simulink model "sensor_fusion"  (R2026a)
settings: Solver=ode1  StopTime=inf  FixedStep=1/60  EnableMultiTasking=on
model workspace (MAT data in the model file):
  downCamStepSize = Simulink.Parameter
  downCamStepSize.Value = Simulink.data.Expression
  downCamStepSize.Value.ExpressionString = "qc_get_step_size*ceil(1/60/qc_get_step_size)"
  downCamStepSize.Complexity = 'real'
  downCamStepSize.Dimensions = -1
  downCamStepSize.DataType = 'auto'
  lidarStepSize = Simulink.Parameter
  lidarStepSize.Value = Simulink.data.Expression
  lidarStepSize.Value.ExpressionString = "qc_get_step_size*ceil(1/5/qc_get_step_size)"
  lidarStepSize.Complexity = 'real'
  lidarStepSize.Dimensions = -1
  lidarStepSize.DataType = 'auto'
  mainStepSize = Simulink.Parameter
  mainStepSize.Value = Simulink.data.Expression
  mainStepSize.Value.ExpressionString = "qc_get_step_size"
  mainStepSize.Complexity = 'real'
  mainStepSize.Dimensions = -1
  mainStepSize.DataType = 'auto'
  mode = Simulink.Parameter
  mode.Value = 1
  mode.Complexity = 'real'
  mode.Dimensions = [1 1]
  mode.Description = '0 - education speeds via wheel speed commands
    | 1 - education speeds via body speed commands
    | 2 - research speeds via wheel speed commands
    | 3 - research speeds via body speed commands'
  mode.DataType = 'auto'
  realSenseStepSize = Simulink.Parameter
  realSenseStepSize.Value = Simulink.data.Expression
  realSenseStepSize.Value.ExpressionString = "qc_get_step_size*ceil(1/30/qc_get_step_size)"
  realSenseStepSize.Complexity = 'real'
  realSenseStepSize.Dimensions = -1
  realSenseStepSize.DataType = 'auto'
undefined symbols (not defined in the file): Point
libraries: quarc_library x21, simulink x2
settings Model: SimulationMode=external  ExtModeTrigDuration=10000  Creator=mbohra  LastModifiedBy=rdu
settings SolverCC: PositivePriorityOrder=on
settings DebuggingCC: ParameterPrecisionLossMsg=none
settings HardwareCC: ProdBitPerLong=64.0  ProdLargestAtomicInteger=LongLong  ProdLargestAtomicFloat=Double  ProdHWDeviceType=ARM Compatible->ARM 64-bit (LP64)
settings RTWCC: SystemTargetFile=quarc_linux_qbot_platform.tlc  TemplateMakefile=quarc_default_tmf  Toolchain=QUARC linux_qbot_platform | gmake (64-bit Windows)  BuildConfiguration=Faster Runs  Description=QUARC Linux QBot Platform Target Using Toolchain
settings STFCustomTargetCC: SystemTargetFile=quarc_linux_qbot_platform.tlc  MultiwordLength=2048.0  ConcurrentExecutionCompliant=on  UseToolchainInfoCompliant=on  StripSymbols=off  MinimumThreadPriority=20.0
settings GRTTargetCC: ExtMode=on  ExtModeMexFile=quarc_comm  ExtModeMexArgs='-w -d /tmp -uri %u','tcpip://192.168.5.3:17001'  ParMdlRefBuildCompliant=off  CompOptLevelCompliant=off  CombineOutputUpdateFcns=off  MatFileLogging=off  CPPClassGenCompliant=off  GRTInterface=on
settings ConfigComp: CovMetricSettings=dswe

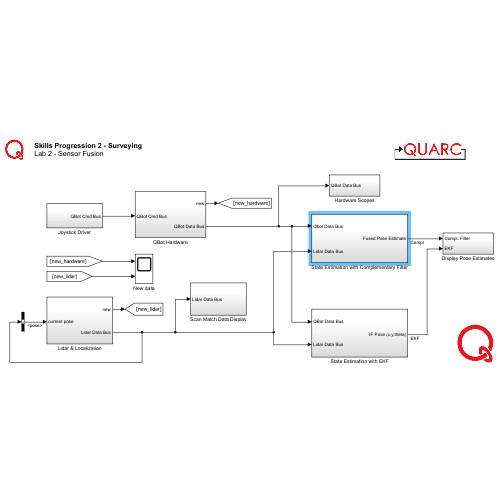
[thumbnail: Simulink's stored preview of the top-level diagram]
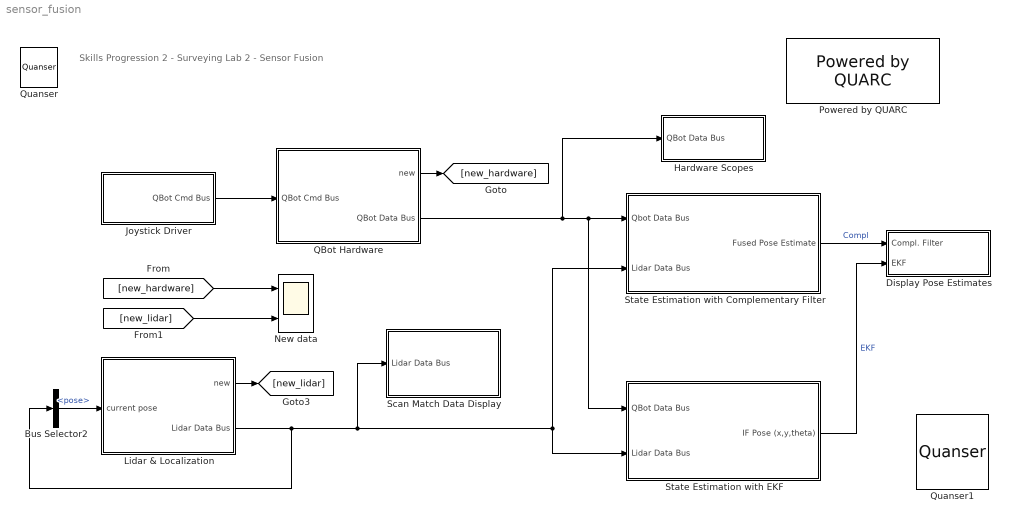
== system sensor_fusion ==
  note: Skills Progression 2 - Surveying
      | Lab 2 - Sensor Fusion
  Bus Selector2 : BusSelector  OutputSignals=pose
  Display Pose Estimates : Subsystem
  Hardware Scopes : Subsystem
  Joystick Driver : Subsystem
  Lidar & Localization : Subsystem
  New data : Scope  NumInputPorts=2
      settings: Title=Hardware Data New?  ActiveDisplayYMinimum=0.9  ActiveDisplayYMaximum=1.1  DataLoggingDecimation=10  DataLoggingVariableName=ScopeData2
  Powered by QUARC : quarc_library/Logos/Powered by QUARC
  QBot Hardware : Subsystem
  Quanser : quarc_library/Logos/Quanser
  Quanser1 : quarc_library/Logos/Quanser
  Scan Match Data Display : Subsystem
  State Estimation with Complementary Filter : Subsystem
  State Estimation with EKF : Subsystem
  wires:
  QBot Hardware/1(new) -> [new_hardware]
  Lidar & Localization/1(new) -> [new_lidar]
  [new_lidar] -> New data/2
  [new_hardware] -> New data/1
  Bus Selector2/1 -> Lidar & Localization/1(current pose)  "<pose>"
  Lidar & Localization/2(Lidar Data Bus) -> State Estimation with EKF/2(Lidar Data Bus), State Estimation with Complementary Filter/2(Lidar Data Bus), Scan Match Data Display/1(Lidar Data Bus), Bus Selector2/1
  Joystick Driver/1(QBot Cmd Bus) -> QBot Hardware/1(QBot Cmd Bus)
  QBot Hardware/2(QBot Data Bus) -> State Estimation with Complementary Filter/1(Qbot Data Bus), State Estimation with EKF/1(QBot Data Bus), Hardware Scopes/1(QBot Data Bus)
  State Estimation with Complementary Filter/1(Fused Pose Estimate) -> Display Pose Estimates/1(Compl. Filter)  "Compl"
  State Estimation with EKF/1(IF Pose (x,y,theta)) -> Display Pose Estimates/2(EKF)  "EKF"

== system sensor_fusion/Display Pose Estimates ==
  Compl. Filter : Inport
  EKF : Inport  Port=2
  Mux : Mux  Inputs=2
  Mux1 : Mux  Inputs=2
  Mux2 : Mux  Inputs=2
  "Pose Estimates " : Scope  NumInputPorts=3
      settings: ActiveDisplayString=3  Title=Theta (rad)  ActiveDisplayYMinimum=-3.7845885644041823  ActiveDisplayYMaximum=8.5346333601811839  DataLoggingVariableName=ScopeData4
  Selector : Selector  InputPortWidth=3  IndexOptions=Index vector (dialog)  Indices=[1]  OutputSizes=1
  Selector1 : Selector  InputPortWidth=3  IndexOptions=Index vector (dialog)  Indices=[1]  OutputSizes=1
  Selector2 : Selector  InputPortWidth=3  IndexOptions=Index vector (dialog)  Indices=[2]  OutputSizes=1
  Selector3 : Selector  InputPortWidth=3  IndexOptions=Index vector (dialog)  Indices=[2]  OutputSizes=1
  Selector4 : Selector  InputPortWidth=3  IndexOptions=Index vector (dialog)  Indices=[3]  OutputSizes=1
  Selector5 : Selector  InputPortWidth=3  IndexOptions=Index vector (dialog)  Indices=[3]  OutputSizes=1
  wires:
  Compl. Filter/1 -> Selector4/1, Selector2/1, Selector/1
  Mux/1 -> "Pose Estimates "/1
  Selector/1 -> Mux/1  "Compl"
  EKF/1 -> Selector5/1, Selector3/1, Selector1/1
  Selector1/1 -> Mux/2  "EKF"
  Selector2/1 -> Mux1/1  "Compl"
  Selector3/1 -> Mux1/2  "EKF"
  Selector5/1 -> Mux2/2  "EKF"
  Selector4/1 -> Mux2/1  "Compl"
  Mux1/1 -> "Pose Estimates "/2
  Mux2/1 -> "Pose Estimates "/3

== system sensor_fusion/Hardware Scopes ==
  QBot Data Bus : Inport
  Accelerometer : Scope  Commented=on
      settings: ActiveDisplayYMinimum=-1.32758  ActiveDisplayYMaximum=11.23  DataLoggingVariableName=ScopeData9
  Battery Sense : Scope  Commented=on
      settings: ActiveDisplayYMinimum=12.81161  ActiveDisplayYMaximum=12.96349  DataLoggingVariableName=ScopeData10
  Bus Selector : BusSelector  OutputSignals=Wheel position (rad) [2],Wheel Speeds (rad/s) [2],Motor Cmd (Volts) [2],Acceleration (m/s/s) [3],Gyroscope (rad/s) [3],Current (Amps) [2],Battery (Volts)
  Cmd Voltage : Scope  Commented=on
      settings: ActiveDisplayYMinimum=-1  ActiveDisplayYMaximum=1  DataLoggingVariableName=ScopeData11
  Current Sense : Scope  Commented=on
      settings: ActiveDisplayYMinimum=-0.05029  ActiveDisplayYMaximum=0.45265  DataLoggingVariableName=ScopeData12
  Encoder : Scope  Commented=on
      settings: ActiveDisplayYMinimum=-23.46955  ActiveDisplayYMaximum=23.65434  DataLoggingVariableName=ScopeData13
  Gyroscope : Scope  Commented=on
      settings: ActiveDisplayYMinimum=-0.40322  ActiveDisplayYMaximum=1.99912  DataLoggingVariableName=ScopeData14
  Tachometer : Scope  Commented=on
      settings: ActiveDisplayYMinimum=-11.69986  ActiveDisplayYMaximum=11.67552  DataLoggingVariableName=ScopeData15
  wires:
  Bus Selector/6 -> Current Sense/1  "<Current (Amps) [2]>"
  QBot Data Bus/1 -> Bus Selector/1
  Bus Selector/3 -> Cmd Voltage/1  "<Motor Cmd (Volts) [2]>"
  Bus Selector/7 -> Battery Sense/1  "<Battery (Volts)>"
  Bus Selector/4 -> Accelerometer/1  "<Acceleration (m/s/s) [3]>"
  Bus Selector/1 -> Encoder/1  "<Wheel position (rad) [2]>"
  Bus Selector/2 -> Tachometer/1  "<Wheel Speeds (rad/s) [2]>"
  Bus Selector/5 -> Gyroscope/1  "<Gyroscope (rad/s) [3]>"

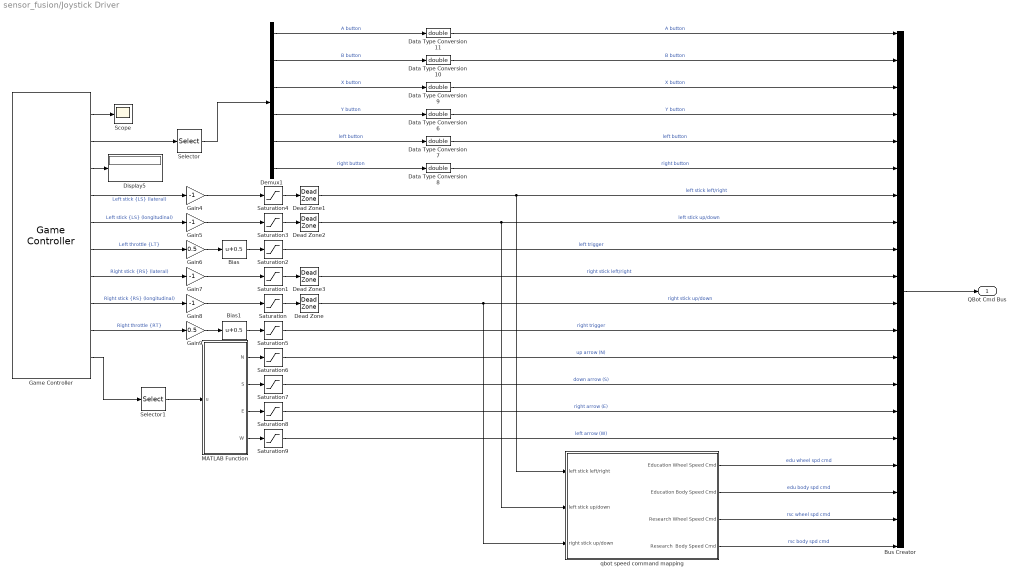
== system sensor_fusion/Joystick Driver ==
  Bias : Bias  Bias=0.5  SaturateOnIntegerOverflow=off
  Bias1 : Bias  Bias=0.5  SaturateOnIntegerOverflow=off
  Bus Creator : BusCreator  Inputs=20
  Data Type Conversion{6..11} (6 alike) : DataTypeConversion  OutDataTypeStr=double  SaturateOnIntegerOverflow=off  RndMeth=Floor
  Dead Zone{,1..3} (4 alike) : DeadZone  LowerValue=-0.05  UpperValue=0.05
  Demux1 : Demux  Outputs=6
  Display5 : Display
  Gain{4..5,7..8} (4 alike) : Gain  Gain=-1
  Gain6 : Gain  Gain=0.5
  Gain9 : Gain  Gain=0.5
  Game Controller : quarc_library/Devices/Peripherals/Target/Game Controller  controller=1  buffer_size=12  deadzone=[]  saturation=[]  sample_time=qc_get_step_size  auto_center=off  enabled=on
      settings: SourceProductName=QUARC Targets
  MATLAB Function : MATLAB Function  TreatAsAtomicUnit=on
  Saturation{,1,3..4} (4 alike) : Saturate  UpperLimit=1  LowerLimit=-1
  Saturation{2,5..9} (6 alike) : Saturate  UpperLimit=1  LowerLimit=0
  Scope : Scope
      settings: ActiveDisplayYMinimum=-1  ActiveDisplayYMaximum=1
  Selector : Selector  InputPortWidth=32  IndexOptions=Index vector (dialog)  Indices=[1:6]  OutputSizes=1
  Selector1 : Selector  InputPortWidth=4  IndexOptions=Index vector (dialog)  Indices=1  OutputSizes=1
  qbot speed command mapping : Subsystem
  QBot Cmd Bus : Outport
  wires:
  Game Controller/1 -> Scope/1
  Game Controller/2 -> Selector/1
  Game Controller/3 -> Display5/1
  Game Controller/4 -> Gain4/1  "Left stick {LS} (lateral)"
  Game Controller/5 -> Gain5/1  "Left stick {LS} (longitudinal)"
  Game Controller/6 -> Gain6/1  "Left throttle {LT}"
  Game Controller/7 -> Gain7/1  "Right stick {RS} (lateral)"
  Game Controller/8 -> Gain8/1  "Right stick {RS} (longitudinal)"
  Game Controller/9 -> Gain9/1  "Right throttle {RT}"
  Game Controller/10 -> Selector1/1
  Selector/1 -> Demux1/1
  Selector1/1 -> MATLAB Function/1(u)
  Gain6/1 -> Bias/1
  Gain9/1 -> Bias1/1
  Gain8/1 -> Saturation/1
  Gain7/1 -> Saturation1/1
  Gain5/1 -> Saturation3/1
  Gain4/1 -> Saturation4/1
  Bias/1 -> Saturation2/1
  Bias1/1 -> Saturation5/1
  Saturation4/1 -> Dead Zone1/1
  Saturation3/1 -> Dead Zone2/1
  Saturation1/1 -> Dead Zone3/1
  Saturation/1 -> Dead Zone/1
  MATLAB Function/1(N) -> Saturation6/1
  MATLAB Function/2(S) -> Saturation7/1
  MATLAB Function/3(E) -> Saturation8/1
  MATLAB Function/4(W) -> Saturation9/1
  Demux1/5 -> Data Type Conversion7/1  "left button"
  Demux1/6 -> Data Type Conversion8/1  "right button"
  Dead Zone/1 -> qbot speed command mapping/3(right stick up/down), Bus Creator/11  "right stick up/down"
  Dead Zone1/1 -> qbot speed command mapping/1(left stick left/right), Bus Creator/7  "left stick left/right"
  Demux1/4 -> Data Type Conversion6/1  "Y button"
  Demux1/3 -> Data Type Conversion9/1  "X button"
  Demux1/2 -> Data Type Conversion10/1  "B button"
  Demux1/1 -> Data Type Conversion11/1  "A button"
  Dead Zone2/1 -> qbot speed command mapping/2(left stick up/down), Bus Creator/8  "left stick up/down"
  Saturation6/1 -> Bus Creator/13  "up arrow (N)"
  Saturation7/1 -> Bus Creator/14  "down arrow (S)"
  Saturation8/1 -> Bus Creator/15  "right arrow (E)"
  Saturation9/1 -> Bus Creator/16  "left arrow (W)"
  qbot speed command mapping/1(Education Wheel Speed Cmd) -> Bus Creator/17  "edu wheel spd cmd"
  qbot speed command mapping/2(Education Body Speed Cmd) -> Bus Creator/18  "edu body spd cmd"
  qbot speed command mapping/3(Research Wheel Speed Cmd) -> Bus Creator/19  "rsc wheel spd cmd"
  qbot speed command mapping/4(Research  Body Speed Cmd) -> Bus Creator/20  "rsc body spd cmd"
  Saturation2/1 -> Bus Creator/9  "left trigger"
  Dead Zone3/1 -> Bus Creator/10  "right stick left/right"
  Saturation5/1 -> Bus Creator/12  "right trigger"
  Bus Creator/1 -> QBot Cmd Bus/1
  Data Type Conversion6/1 -> Bus Creator/4  "Y button"
  Data Type Conversion8/1 -> Bus Creator/6  "right button"
  Data Type Conversion7/1 -> Bus Creator/5  "left button"
  Data Type Conversion9/1 -> Bus Creator/3  "X button"
  Data Type Conversion10/1 -> Bus Creator/2  "B button"
  Data Type Conversion11/1 -> Bus Creator/1  "A button"

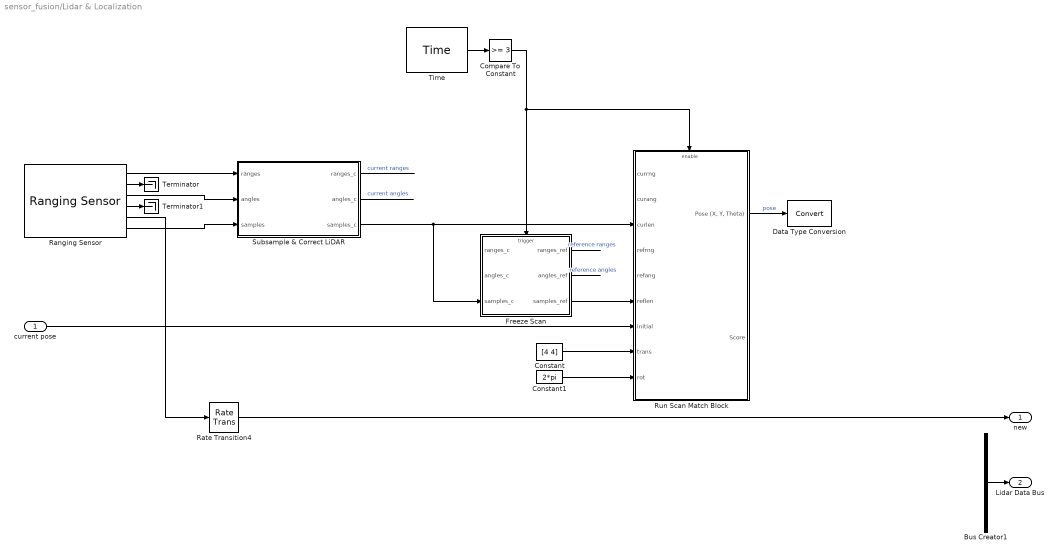
== system sensor_fusion/Lidar & Localization ==
  current pose : Inport
  Bus Creator1 : BusCreator  Inputs=6
  Compare To Constant : simulink/Logic and Bit Operations/Compare To Constant  relop=>=  const=3  OutDataTypeStr=boolean
  Constant : Constant  Value=[4 4]
  Constant1 : Constant  Value=2*pi
  Data Type Conversion : DataTypeConversion  SaturateOnIntegerOverflow=off  RndMeth=Floor
  Freeze Scan : Subsystem  TreatAsAtomicUnit=on
  Ranging Sensor : quarc_library/Devices/Third-Party/Sensors/Ranging Sensor  sensor_type=Leishen M10P LIDAR  uri=serial://localhost:0?device='/dev/lidar',baud='512000',word='8',parity='none',stop='1',flow='none'  ranging_distance=Short  timing_budget=0.033  measurement_period=0.0005  output_mode=Fixed-size output  samples_per_revolution=1680  max_distance=0.050  max_angle=5  sample_time=lidarStepSize  show_versions=off  active=on
      settings: SourceProductName=QUARC Targets
  Rate Transition4 : RateTransition
  Run Scan Match Block : Subsystem
  Subsample & Correct LiDAR : Subsystem
  Terminator : Terminator
  Terminator1 : Terminator
  Time : quarc_library/Sources/Time/Time  time_source=Wall clock  sample_time=lidarStepSize
  new : Outport
  Lidar Data Bus : Outport  Port=2
  wires:
  Ranging Sensor/5 -> Rate Transition4/1
  Rate Transition4/1 -> new/1
  Ranging Sensor/2 -> Terminator/1
  Ranging Sensor/4 -> Terminator1/1
  Compare To Constant/1 -> Run Scan Match Block/Enable, Freeze Scan/Trigger
  Run Scan Match Block/1("Pose (X, Y, Theta)") -> Data Type Conversion/1  "pose"
  Freeze Scan/3(samples_ref) -> Run Scan Match Block/6(reflen)
  Time/1 -> Compare To Constant/1
  Bus Creator1/1 -> Lidar Data Bus/1
  current pose/1 -> Run Scan Match Block/7(initial)
  Constant/1 -> Run Scan Match Block/8(trans)
  Constant1/1 -> Run Scan Match Block/9(rot)
  Subsample & Correct LiDAR/3(samples_c) -> Run Scan Match Block/3(curlen), Freeze Scan/3(samples_c)
  Ranging Sensor/1 -> Subsample & Correct LiDAR/1(ranges)
  Ranging Sensor/3 -> Subsample & Correct LiDAR/2(angles)
  Ranging Sensor/6 -> Subsample & Correct LiDAR/3(samples)
  Subsample & Correct LiDAR/1(ranges_c) -> ?  "current ranges"
  Subsample & Correct LiDAR/2(angles_c) -> ?  "current angles"
  ? -> Freeze Scan/1(ranges_c)
  ? -> Freeze Scan/2(angles_c)
  ? -> Bus Creator1/5  "pose"
  ? -> Bus Creator1/6  "score"
  ? -> Bus Creator1/3  "reference ranges"
  ? -> Bus Creator1/4  "reference angles"
  ? -> Bus Creator1/1  "current ranges"
  ? -> Bus Creator1/2  "current angles"
  Freeze Scan/1(ranges_ref) -> ?  "reference ranges"
  Freeze Scan/2(angles_ref) -> ?  "reference angles"

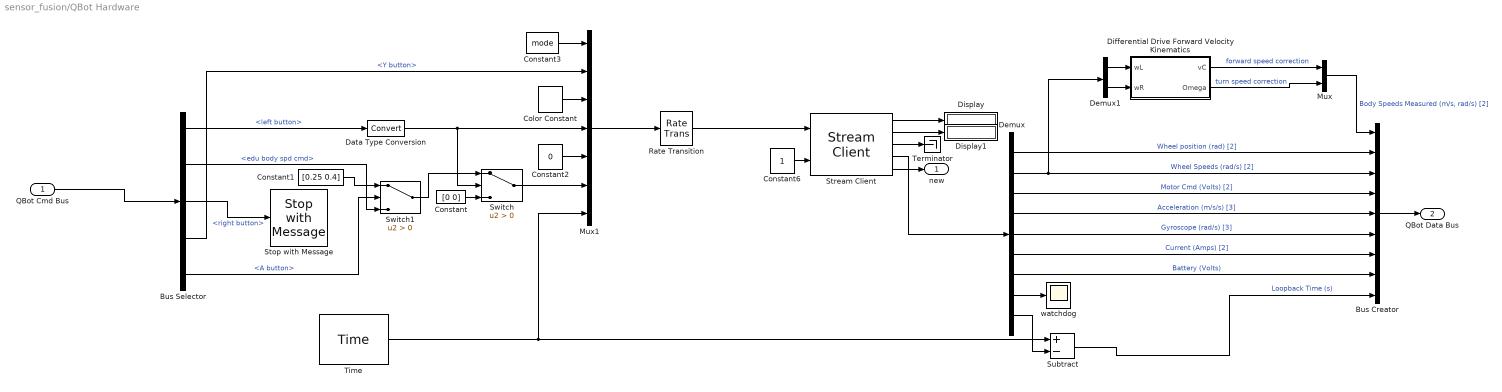
== system sensor_fusion/QBot Hardware ==
  QBot Cmd Bus : Inport
  Bus Creator : BusCreator  Inputs=9
  Bus Selector : BusSelector  OutputSignals=left button,edu body spd cmd,right button,Y button,A button
  Color Constant : quarc_library/Sources/Signals/Color Constant  color=[1 0 1]
      settings: SourceProductName=QUARC Targets
  Constant : Constant  Value=[0 0]
  Constant1 : Constant  Value=[0.25 0.4]
  Constant2 : Constant  Value=0
  Constant3 : Constant  Value=mode
  Constant6 : Constant
  Data Type Conversion : DataTypeConversion  SaturateOnIntegerOverflow=off  RndMeth=Floor
  Demux : Demux  Outputs=[2 2 2 3 3 2 1 1 1]
  Demux1 : Demux  Outputs=2
  Differential Drive Forward Velocity Kinematics : MATLAB Function  TreatAsAtomicUnit=on
  Display : Display
  Display1 : Display
  Mux : Mux  Inputs=2
  Mux1 : Mux  Inputs=7
  Rate Transition : RateTransition
  Stop with Message : quarc_library/Sinks/Error Handling/Stop with Message  message_type=Fixed error message  message_icon=Information  message=Operator: Emergency Stop
  Stream Client : quarc_library/Communications/Basic/Stream Client  uri_source=Specify via dialog (do not evaluate)  uri=tcpip://localhost:18888  send_buffer_size=1460  receive_buffer_size=1460  byte_order=little endian (Intel - LSB first)  optimization=Minimum latency  send_options=Send most recent data  receive_options=Receive most recent data  default_value=zeros(17,1)  sample_time=qc_get_step_size  active=off  implementation=Use blocking I/O in a separate thread  send_fifo_size=1000  receive_fifo_size=1000  send_priority=0  receive_priority=0  send_dimensions=off  receive_dimensions=off  max_dimensions=-1  data_type=Inherited via back propagation  type_expr=BusObject
      settings: AttributesFormatString="\"tcpip://localhost:18888\""
  Subtract : Sum  Inputs=+-
  Switch : Switch  Criteria=u2 > Threshold  SaturateOnIntegerOverflow=off  InputSameDT=off
  Switch1 : Switch  Criteria=u2 > Threshold  SaturateOnIntegerOverflow=off  InputSameDT=off
  Terminator : Terminator
  Time : quarc_library/Sources/Time/Time  time_source=Wall clock  sample_time=qc_get_step_size
  watchdog : Scope
  new : Outport
  QBot Data Bus : Outport  Port=2
  wires:
  Constant3/1 -> Mux1/1
  Stream Client/3 -> Terminator/1
  Bus Selector/2 -> Switch1/3  "<edu body spd cmd>"
  Stream Client/1 -> Display/1
  Constant6/1 -> Stream Client/2
  Stream Client/2 -> Display1/1
  Color Constant/1 -> Mux1/3
  Demux/3 -> Bus Creator/4  "Motor Cmd (Volts) [2]"
  Mux1/1 -> Rate Transition/1
  Stream Client/4 -> Demux/1
  Demux/1 -> Bus Creator/2  "Wheel position (rad) [2]"
  Stream Client/5 -> new/1
  Demux/7 -> Bus Creator/8  "Battery (Volts)"
  Demux/5 -> Bus Creator/6  "Gyroscope (rad/s) [3]"
  Demux/6 -> Bus Creator/7  "Current (Amps) [2]"
  Demux/9 -> Subtract/2
  Constant2/1 -> Mux1/5
  Demux/4 -> Bus Creator/5  "Acceleration (m/s/s) [3]"
  Time/1 -> Subtract/1, Mux1/7
  Bus Creator/1 -> QBot Data Bus/1
  Subtract/1 -> Bus Creator/9  "Loopback Time (s)"
  Demux/8 -> watchdog/1
  QBot Cmd Bus/1 -> Bus Selector/1
  Bus Selector/3 -> Stop with Message/1  "<right button>"
  Bus Selector/1 -> Data Type Conversion/1  "<left button>"
  Data Type Conversion/1 -> Mux1/4, Switch/2
  Bus Selector/4 -> Mux1/2  "<Y button>"
  Demux/2 -> Bus Creator/3, Demux1/1  "Wheel Speeds (rad/s) [2]"
  Demux1/2 -> Differential Drive Forward Velocity Kinematics/2(wR)
  Demux1/1 -> Differential Drive Forward Velocity Kinematics/1(wL)
  Differential Drive Forward Velocity Kinematics/2(Omega) -> Mux/2  "turn speed correction"
  Differential Drive Forward Velocity Kinematics/1(vC) -> Mux/1  "forward speed correction"
  Mux/1 -> Bus Creator/1  "Body Speeds Measured (m/s, rad/s) [2]"
  Rate Transition/1 -> Stream Client/1
  Switch/1 -> Mux1/6
  Constant1/1 -> Switch1/1
  Bus Selector/5 -> Switch1/2  "<A button>"
  Constant/1 -> Switch/3
  Switch1/1 -> Switch/1

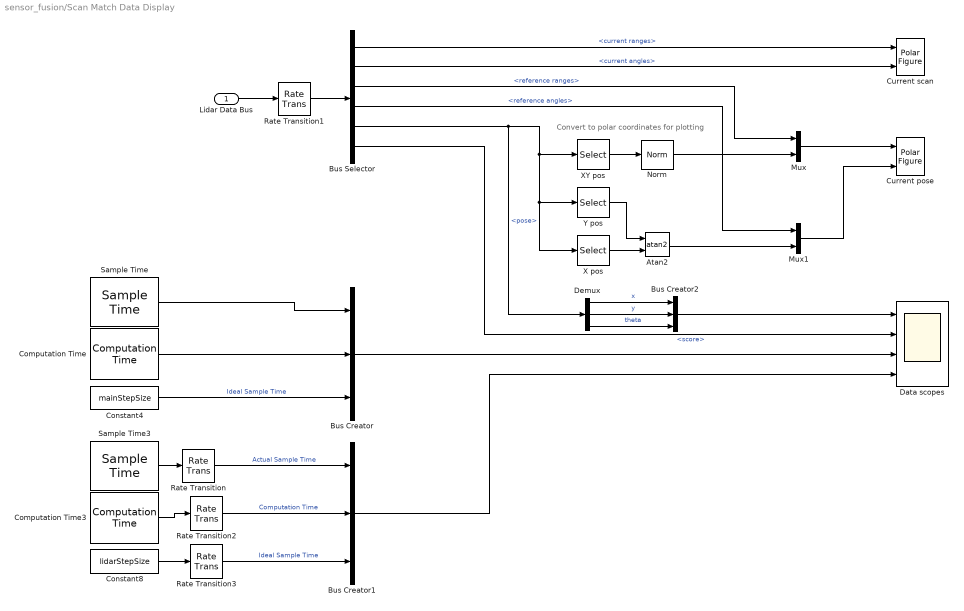
== system sensor_fusion/Scan Match Data Display ==
  note: Convert to polar coordinates for plotting
  Lidar Data Bus : Inport
  Atan2 : Trigonometry  Operator=atan2
  Bus Creator : BusCreator  Inputs=3
  Bus Creator1 : BusCreator  Inputs=3
  Bus Creator2 : BusCreator  Inputs=3
  Bus Selector : BusSelector  OutputSignals=current ranges,current angles,reference ranges,reference angles,pose,score
  Computation Time : quarc_library/Sources/Time/Computation Time  sample_time=mainStepSize  use_model=on  use_cpu_time=off
  Computation Time3 : quarc_library/Sources/Time/Computation Time  sample_time=lidarStepSize  use_model=on  use_cpu_time=off
  Constant4 : Constant  Value=mainStepSize
  Constant8 : Constant  Value=lidarStepSize
  Current pose : quarc_library/Sinks/Figures/Polar Figure  figure_mode=Use figure window  figure_tag=figure1  axes_tag=axes1  plot_mode=Frame-based  minimum_rho=0  maximum_rho=4  minimum_theta=0  maximum_theta=360  zero_location=right  direction=counterclockwise  buffer_size=421  update_rate=1  sample_time=-1  initial_position="841  452  616  412"  initial_visibility=off  line1_style=None  line1_width=0.5  line1_color=[1 0 0]  marker1=Point (.)  marker1_size=6  marker1_edge_color=[1 0 0]  marker1_face_color=[1 0 0]  line2_style=None  line2_width=0.5  line2_color=[0.85098 0.32549 0.0980392]  marker2=Cross (x)  marker2_size=6  marker2_edge_color=[0.85098 0.32549 0.0980392]  marker2_face_color=[0.85098 0.32549 0.0980392]  line3_style=Solid line (-)  line3_width=0.5  line3_color=[0.929412 0.694118 0.12549]  marker3=None  marker3_size=6  marker3_edge_color=[0.929412 0.694118 0.12549]  marker3_face_color=[0.929412 0.694118 0.12549]  line4_style=Solid line (-)  line4_width=0.5  line4_color=[0.494118 0.184314 0.556863]  marker4=None  marker4_size=6  marker4_edge_color=[0.494118 0.184314 0.556863]  marker4_face_color=[0.494118 0.184314 0.556863]  line5_style=Solid line (-)  line5_width=0.5  line5_color=[0.466667 0.67451 0.188235]  marker5=None  marker5_size=6  marker5_edge_color=[0.466667 0.67451 0.188235]  marker5_face_color=[0.466667 0.67451 0.188235]
      settings: SourceProductName=QUARC Targets
  Current scan : quarc_library/Sinks/Figures/Polar Figure  figure_mode=Use figure window  figure_tag=figure1  axes_tag=axes1  plot_mode=Frame-based  minimum_rho=0  maximum_rho=4  minimum_theta=0  maximum_theta=360  zero_location=right  direction=counterclockwise  buffer_size=2  update_rate=1  sample_time=-1  initial_position="60    84  1189   906"  initial_visibility=off  line1_style=None  line1_width=0.5  line1_color=[1 0 0]  marker1=Point (.)  marker1_size=6  marker1_edge_color=[1 0 0]  marker1_face_color=[1 0 0]  line2_style=Solid line (-)  line2_width=0.5  line2_color=[0.85098 0.32549 0.0980392]  marker2=None  marker2_size=6  marker2_edge_color=[0.85098 0.32549 0.0980392]  marker2_face_color=[0.85098 0.32549 0.0980392]  line3_style=Solid line (-)  line3_width=0.5  line3_color=[0.929412 0.694118 0.12549]  marker3=None  marker3_size=6  marker3_edge_color=[0.929412 0.694118 0.12549]  marker3_face_color=[0.929412 0.694118 0.12549]  line4_style=Solid line (-)  line4_width=0.5  line4_color=[0.494118 0.184314 0.556863]  marker4=None  marker4_size=6  marker4_edge_color=[0.494118 0.184314 0.556863]  marker4_face_color=[0.494118 0.184314 0.556863]  line5_style=Solid line (-)  line5_width=0.5  line5_color=[0.466667 0.67451 0.188235]  marker5=None  marker5_size=6  marker5_edge_color=[0.466667 0.67451 0.188235]  marker5_face_color=[0.466667 0.67451 0.188235]
      settings: SourceProductName=QUARC Targets
  Data scopes : Scope  NumInputPorts=4
      settings: ActiveDisplayString=4  Title=Lidar Timing  ActiveDisplayYMinimum=-0.0634349307717868  ActiveDisplayYMaximum=0.23596947906500806  DataLoggingDecimation=10  DataLoggingVariableName=ScopeData3
  Demux : Demux  Outputs=3
  Mux : Mux  Inputs=2
  Mux1 : Mux  Inputs=2
  Norm : quarc_library/Math Operations/Vectors/Norm
      settings: SourceProductName=QUARC Targets
  Rate Transition{,1..3} (4 alike) : RateTransition
  Sample Time : quarc_library/Sources/Time/Sample Time  Priority=-99  sample_time=mainStepSize
  Sample Time3 : quarc_library/Sources/Time/Sample Time  Priority=-99  sample_time=lidarStepSize
  X pos : Selector  InputPortWidth=3  IndexOptions=Index vector (dialog)  Indices=[1]  OutputSizes=1
  "XY pos " : Selector  InputPortWidth=3  IndexOptions=Index vector (dialog)  Indices=[1 2]  OutputSizes=1
  Y pos : Selector  InputPortWidth=3  IndexOptions=Index vector (dialog)  Indices=2  OutputSizes=1
  wires:
  Bus Selector/5 -> Demux/1, X pos/1, Y pos/1, "XY pos "/1  "<pose>"
  "XY pos "/1 -> Norm/1
  Y pos/1 -> Atan2/1
  X pos/1 -> Atan2/2
  Atan2/1 -> Mux1/2
  Norm/1 -> Mux/2
  Lidar Data Bus/1 -> Rate Transition1/1
  Bus Selector/1 -> Current scan/1  "<current ranges>"
  Bus Selector/2 -> Current scan/2  "<current angles>"
  Bus Selector/3 -> Mux/1  "<reference ranges>"
  Bus Selector/4 -> Mux1/1  "<reference angles>"
  Bus Selector/6 -> Data scopes/2  "<score>"
  Mux1/1 -> Current pose/2
  Mux/1 -> Current pose/1
  Sample Time3/1 -> Rate Transition/1
  Constant8/1 -> Rate Transition3/1
  Computation Time/1 -> Bus Creator/2
  Computation Time3/1 -> Rate Transition2/1
  Sample Time/1 -> Bus Creator/1
  Constant4/1 -> Bus Creator/3  "Ideal Sample Time"
  Rate Transition1/1 -> Bus Selector/1
  Bus Creator1/1 -> Data scopes/4
  Demux/1 -> Bus Creator2/1  "x"
  Demux/2 -> Bus Creator2/2  "y"
  Demux/3 -> Bus Creator2/3  "theta"
  Bus Creator2/1 -> Data scopes/1
  Rate Transition/1 -> Bus Creator1/1  "Actual Sample Time"
  Rate Transition2/1 -> Bus Creator1/2  "Computation Time"
  Rate Transition3/1 -> Bus Creator1/3  "Ideal Sample Time"
  Bus Creator/1 -> Data scopes/3

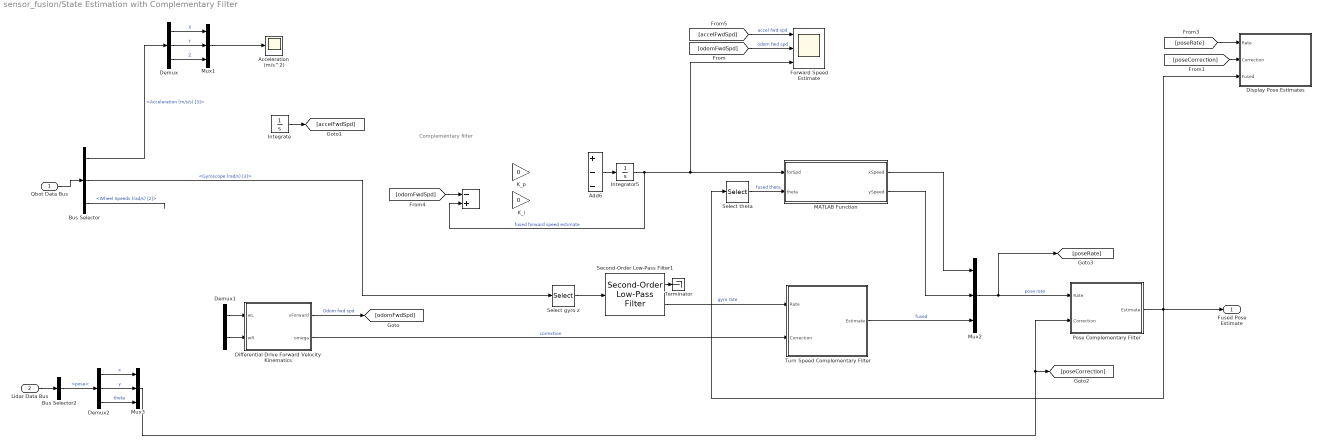
== system sensor_fusion/State Estimation with Complementary Filter ==
  note: Complementary filter
  Qbot Data Bus : Inport
  Lidar Data Bus : Inport  Port=2
  " " : Sum  Inputs=-+
  Acceleration (m/s^2) : Scope
      settings: TimeSpan=10  ActiveDisplayYMinimum=-0.21830889279586507  ActiveDisplayYMaximum=0.25440172069065836  DataLoggingVariableName=ScopeData10
  Add6 : Sum  Inputs=+--
  Bus Selector : BusSelector  OutputSignals=Acceleration (m/s/s) [3],Gyroscope (rad/s) [3],Wheel Speeds (rad/s) [2]
  Bus Selector2 : BusSelector  OutputSignals=pose
  Demux : Demux  Outputs=3
  Demux1 : Demux  Outputs=2
  Demux2 : Demux  Outputs=3
  Differential Drive Forward Velocity Kinematics : MATLAB Function  TreatAsAtomicUnit=on
  Display Pose Estimates : Subsystem
  Forward Speed Estimate : Scope  NumInputPorts=3
      settings: TimeSpan=10  ActiveDisplayYMinimum=-0.21338677605532697  ActiveDisplayYMaximum=0.24552368348060344  DataLoggingVariableName=ScopeData9
  Integrate : Integrator
  Integrator5 : Integrator
  K_i : Gain  Gain=0
  K_p : Gain  Gain=0
  MATLAB Function : MATLAB Function  TreatAsAtomicUnit=on
  Mux1 : Mux  Inputs=3
  Mux2 : Mux  Inputs=3
  Mux3 : Mux  Inputs=3
  Pose Complementary Filter : Subsystem
  Second-Order Low-Pass Filter1 : quarc_library/Continuous/Second-Order Low-Pass Filter  params_source=Internal (dialog parameters)  input_width=10  input_zeta=1  input_init=0
  Select gyro z : Selector  InputPortWidth=3  IndexOptions=Index vector (dialog)  Indices=[3]  OutputSizes=1
  Select theta : Selector  InputPortWidth=3  IndexOptions=Index vector (dialog)  Indices=3  OutputSizes=1
  Terminator : Terminator
  Turn Speed Complementary Filter : Subsystem
  Fused Pose Estimate : Outport
  wires:
  Qbot Data Bus/1 -> Bus Selector/1
  Bus Selector/1 -> Demux/1  "<Acceleration (m/s/s) [3]>"
  Demux1/1 -> Differential Drive Forward Velocity Kinematics/1(wL)
  Demux1/2 -> Differential Drive Forward Velocity Kinematics/2(wR)
  Add6/1 -> Integrator5/1
  Demux/1 -> Mux1/1  "X"
  Demux/2 -> Mux1/2  "Y"
  Demux/3 -> Mux1/3  "Z"
  Mux1/1 -> Acceleration (m/s^2)/1
  [odomFwdSpd] -> Forward Speed Estimate/2  "odom fwd spd"
  [accelFwdSpd] -> Forward Speed Estimate/1  "accel fwd spd"
  Mux2/1 -> Pose Complementary Filter/1(Rate), [poseRate]  "pose rate"
  MATLAB Function/2(ySpeed) -> Mux2/2
  Integrator5/1 -> MATLAB Function/1(forSpd), Forward Speed Estimate/3, " "/2  "fused forward speed estimate"
  MATLAB Function/1(xSpeed) -> Mux2/1
  Pose Complementary Filter/1(Estimate) -> Select theta/1, Fused Pose Estimate/1, Display Pose Estimates/3(Fused)
  Select theta/1 -> MATLAB Function/2(theta)  "fused theta"
  Second-Order Low-Pass Filter1/2 -> Turn Speed Complementary Filter/1(Rate)  "gyro rate"
  Second-Order Low-Pass Filter1/1 -> Terminator/1
  Integrate/1 -> [accelFwdSpd]
  Select gyro z/1 -> Second-Order Low-Pass Filter1/1
  Differential Drive Forward Velocity Kinematics/2(omega) -> Turn Speed Complementary Filter/2(Correction)  "correction"
  Mux3/1 -> Pose Complementary Filter/2(Correction), [poseCorrection]
  Bus Selector/2 -> Select gyro z/1  "<Gyroscope (rad/s) [3]>"
  [odomFwdSpd] -> " "/1
  Differential Drive Forward Velocity Kinematics/1(vForward) -> [odomFwdSpd]  "Odom fwd spd"
  Turn Speed Complementary Filter/1(Estimate) -> Mux2/3  "fused"
  Demux2/1 -> Mux3/1  "x"
  Demux2/2 -> Mux3/2  "y"
  Bus Selector2/1 -> Demux2/1  "<pose>"
  Demux2/3 -> Mux3/3  "theta"
  Lidar Data Bus/1 -> Bus Selector2/1
  [poseCorrection] -> Display Pose Estimates/2(Correction)
  [poseRate] -> Display Pose Estimates/1(Rate)
  ? -> Add6/1, Integrate/1  "fwd accel"
  Bus Selector/3 -> ?  "<Wheel Speeds (rad/s) [2]>"

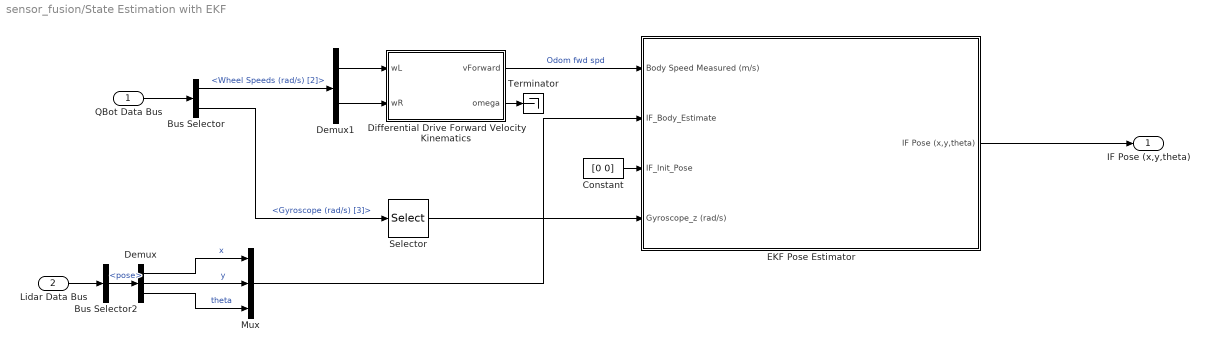
== system sensor_fusion/State Estimation with EKF ==
  QBot Data Bus : Inport
  Lidar Data Bus : Inport  Port=2
  Bus Selector : BusSelector  OutputSignals=Wheel Speeds (rad/s) [2],Gyroscope (rad/s) [3]
  Bus Selector2 : BusSelector  OutputSignals=pose
  Constant : Constant  Value=[0 0]
  Demux : Demux  Outputs=3
  Demux1 : Demux  Outputs=2
  Differential Drive Forward Velocity Kinematics : MATLAB Function  TreatAsAtomicUnit=on
  EKF Pose Estimator : Subsystem
  Mux : Mux  Inputs=3
  Selector : Selector  InputPortWidth=3  IndexOptions=Index vector (dialog)  Indices=[3]  OutputSizes=1
  Terminator : Terminator
  IF Pose (x,y,theta) : Outport
  wires:
  QBot Data Bus/1 -> Bus Selector/1
  Demux1/1 -> Differential Drive Forward Velocity Kinematics/1(wL)
  Demux1/2 -> Differential Drive Forward Velocity Kinematics/2(wR)
  Bus Selector/1 -> Demux1/1  "<Wheel Speeds (rad/s) [2]>"
  Differential Drive Forward Velocity Kinematics/1(vForward) -> EKF Pose Estimator/1(Body Speed Measured (m/s))  "Odom fwd spd"
  Bus Selector/2 -> Selector/1  "<Gyroscope (rad/s) [3]>"
  Selector/1 -> EKF Pose Estimator/4(Gyroscope_z (rad/s))
  EKF Pose Estimator/1(IF Pose (x,y,theta)) -> IF Pose (x,y,theta)/1
  Constant/1 -> EKF Pose Estimator/3(IF_Init_Pose)
  Differential Drive Forward Velocity Kinematics/2(omega) -> Terminator/1
  Demux/1 -> Mux/1  "x"
  Demux/2 -> Mux/2  "y"
  Demux/3 -> Mux/3  "theta"
  Mux/1 -> EKF Pose Estimator/2(IF_Body_Estimate)
  Lidar Data Bus/1 -> Bus Selector2/1
  Bus Selector2/1 -> Demux/1  "<pose>"

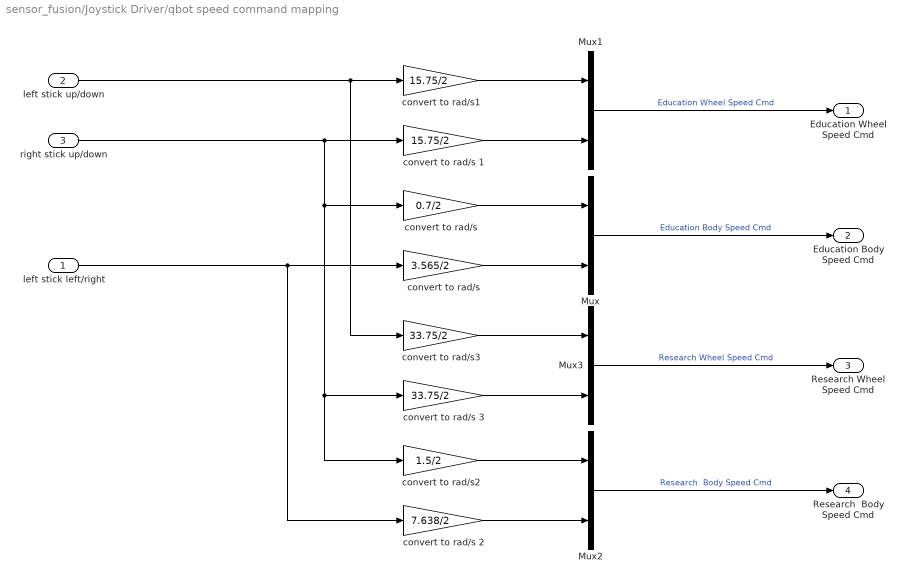
== system sensor_fusion/Joystick Driver/qbot speed command mapping ==
  left stick left/right : Inport
  left stick up/down : Inport  Port=2
  right stick up/down : Inport  Port=3
  Mux{,1..3} (4 alike) : Mux  Inputs=2
  convert to rad/s : Gain  Gain=0.7/2
  "convert to rad/s " : Gain  Gain=3.565/2
  convert to rad/s 1 : Gain  Gain=15.75/2
  convert to rad/s 2 : Gain  Gain=7.638/2
  convert to rad/s 3 : Gain  Gain=33.75/2
  convert to rad/s1 : Gain  Gain=15.75/2
  convert to rad/s2 : Gain  Gain=1.5/2
  convert to rad/s3 : Gain  Gain=33.75/2
  Education Wheel Speed Cmd : Outport
  Education Body Speed Cmd : Outport  Port=2
  Research Wheel Speed Cmd : Outport  Port=3
  Research  Body Speed Cmd : Outport  Port=4
  wires:
  convert to rad/s/1 -> Mux/1
  Mux/1 -> Education Body Speed Cmd/1  "Education Body Speed Cmd"
  left stick left/right/1 -> convert to rad/s 2/1, "convert to rad/s "/1
  convert to rad/s2/1 -> Mux2/1
  left stick up/down/1 -> convert to rad/s3/1, convert to rad/s1/1
  right stick up/down/1 -> convert to rad/s 3/1, convert to rad/s2/1, convert to rad/s/1, convert to rad/s 1/1
  "convert to rad/s "/1 -> Mux/2
  convert to rad/s 3/1 -> Mux3/2
  convert to rad/s3/1 -> Mux3/1
  convert to rad/s 2/1 -> Mux2/2
  convert to rad/s 1/1 -> Mux1/2
  convert to rad/s1/1 -> Mux1/1
  Mux3/1 -> Research Wheel Speed Cmd/1  "Research Wheel Speed Cmd"
  Mux1/1 -> Education Wheel Speed Cmd/1  "Education Wheel Speed Cmd"
  Mux2/1 -> Research  Body Speed Cmd/1  "Research  Body Speed Cmd"

== system sensor_fusion/Lidar & Localization/Freeze Scan ==
  ranges_c : Inport
  angles_c : Inport  Port=2
  samples_c : Inport  Port=3
  Trigger : TriggerPort  VariantControl=(inherit)  InitialTriggerSignalState=zero
  ranges_ref : Outport
  angles_ref : Outport  Port=2
  samples_ref : Outport  Port=3
  wires:
  ranges_c/1 -> ranges_ref/1
  angles_c/1 -> angles_ref/1
  samples_c/1 -> samples_ref/1

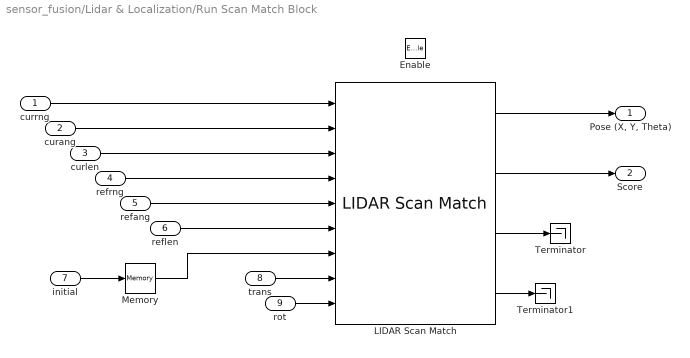
== system sensor_fusion/Lidar & Localization/Run Scan Match Block ==
  currng : Inport
  curang : Inport  Port=2
  curlen : Inport  Port=3
  refrng : Inport  Port=4
  refang : Inport  Port=5
  reflen : Inport  Port=6
  initial : Inport  Port=7
  trans : Inport  Port=8
  rot : Inport  Port=9
  Enable : EnablePort
  LIDAR Scan Match : quarc_library/Image Processing/Generic/LIDAR Scan Match  mode=Fixed input with size  resolution=20  max_range=4  use_initial_pose=on
      settings: SourceProductName=QUARC Targets
  Memory : Memory  InitialCondition=[0 0 0]  InheritSampleTime=on
  Terminator : Terminator
  Terminator1 : Terminator
  "Pose (X, Y, Theta)" : Outport
  Score : Outport  Port=2
  wires:
  refrng/1 -> LIDAR Scan Match/4
  LIDAR Scan Match/2 -> Score/1
  curang/1 -> LIDAR Scan Match/2
  reflen/1 -> LIDAR Scan Match/6
  LIDAR Scan Match/1 -> "Pose (X, Y, Theta)"/1
  refang/1 -> LIDAR Scan Match/5
  currng/1 -> LIDAR Scan Match/1
  curlen/1 -> LIDAR Scan Match/3
  LIDAR Scan Match/3 -> Terminator/1
  LIDAR Scan Match/4 -> Terminator1/1
  Memory/1 -> LIDAR Scan Match/7
  initial/1 -> Memory/1
  trans/1 -> LIDAR Scan Match/8
  rot/1 -> LIDAR Scan Match/9

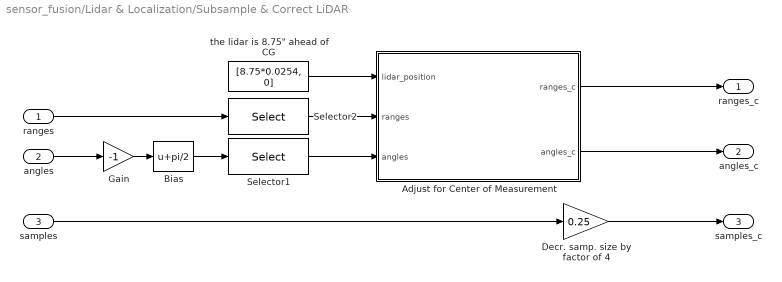
== system sensor_fusion/Lidar & Localization/Subsample & Correct LiDAR ==
  ranges : Inport
  angles : Inport  Port=2
  samples : Inport  Port=3
  Adjust for Center of Measurement : MATLAB Function  TreatAsAtomicUnit=on  SystemSampleTime=lidarStepSize
  Bias : Bias  Bias=pi/2  SaturateOnIntegerOverflow=off
  "Decr. samp. size by factor of 4 " : Gain  Gain=0.25  OutDataTypeStr=int32
  Gain : Gain  Gain=-1
  Selector1 : Selector  InputPortWidth=1680  IndexOptions=Index vector (dialog)  Indices=[1:4:1677]  OutputSizes=1
  Selector2 : Selector  InputPortWidth=1680  IndexOptions=Index vector (dialog)  Indices=[1:4:1677]  OutputSizes=1
  "the lidar is 8.75\" ahead of CG" : Constant  Value=[8.75*0.0254, 0]  SampleTime=lidarStepSize
  ranges_c : Outport
  angles_c : Outport  Port=2
  samples_c : Outport  Port=3
  wires:
  Gain/1 -> Bias/1
  "the lidar is 8.75\" ahead of CG"/1 -> Adjust for Center of Measurement/1(lidar_position)
  samples/1 -> "Decr. samp. size by factor of 4 "/1
  Selector2/1 -> Adjust for Center of Measurement/2(ranges)
  Selector1/1 -> Adjust for Center of Measurement/3(angles)
  ranges/1 -> Selector2/1
  angles/1 -> Gain/1
  Bias/1 -> Selector1/1
  Adjust for Center of Measurement/1(ranges_c) -> ranges_c/1
  Adjust for Center of Measurement/2(angles_c) -> angles_c/1
  "Decr. samp. size by factor of 4 "/1 -> samples_c/1

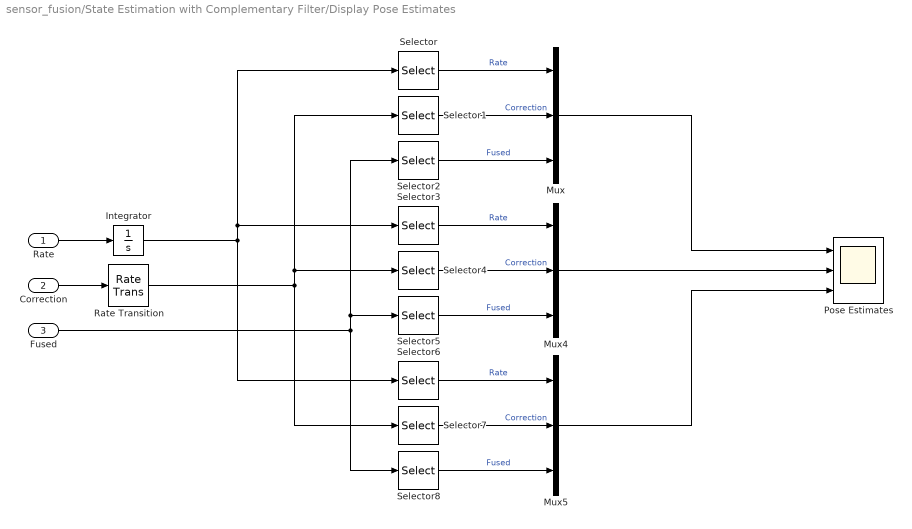
== system sensor_fusion/State Estimation with Complementary Filter/Display Pose Estimates ==
  Rate : Inport
  Correction : Inport  Port=2
  Fused : Inport  Port=3
  Integrator : Integrator
  Mux : Mux  Inputs=3
  Mux4 : Mux  Inputs=3
  Mux5 : Mux  Inputs=3
  Pose Estimates : Scope  NumInputPorts=3
      settings: ActiveDisplayString=3  Title=Theta (rad)  ActiveDisplayYMinimum=-7.2585464207369252  ActiveDisplayYMaximum=7.5280044458771265  DataLoggingVariableName=ScopeData5
  Rate Transition : RateTransition
  Selector : Selector  InputPortWidth=3  IndexOptions=Index vector (dialog)  Indices=[1]  OutputSizes=1
  Selector1 : Selector  InputPortWidth=3  IndexOptions=Index vector (dialog)  Indices=[1]  OutputSizes=1
  Selector2 : Selector  InputPortWidth=3  IndexOptions=Index vector (dialog)  Indices=[1]  OutputSizes=1
  Selector3 : Selector  InputPortWidth=3  IndexOptions=Index vector (dialog)  Indices=[2]  OutputSizes=1
  Selector4 : Selector  InputPortWidth=3  IndexOptions=Index vector (dialog)  Indices=[2]  OutputSizes=1
  Selector5 : Selector  InputPortWidth=3  IndexOptions=Index vector (dialog)  Indices=[2]  OutputSizes=1
  Selector6 : Selector  InputPortWidth=3  IndexOptions=Index vector (dialog)  Indices=[3]  OutputSizes=1
  Selector7 : Selector  InputPortWidth=3  IndexOptions=Index vector (dialog)  Indices=[3]  OutputSizes=1
  Selector8 : Selector  InputPortWidth=3  IndexOptions=Index vector (dialog)  Indices=[3]  OutputSizes=1
  wires:
  Correction/1 -> Rate Transition/1
  Fused/1 -> Selector8/1, Selector5/1, Selector2/1
  Rate Transition/1 -> Selector1/1, Selector4/1, Selector7/1
  Rate/1 -> Integrator/1
  Selector/1 -> Mux/1  "Rate"
  Selector1/1 -> Mux/2  "Correction"
  Selector2/1 -> Mux/3  "Fused"
  Selector3/1 -> Mux4/1  "Rate"
  Selector4/1 -> Mux4/2  "Correction"
  Selector5/1 -> Mux4/3  "Fused"
  Selector6/1 -> Mux5/1  "Rate"
  Selector7/1 -> Mux5/2  "Correction"
  Selector8/1 -> Mux5/3  "Fused"
  Mux/1 -> Pose Estimates/1
  Mux4/1 -> Pose Estimates/2
  Mux5/1 -> Pose Estimates/3
  Integrator/1 -> Selector6/1, Selector/1, Selector3/1

== system sensor_fusion/State Estimation with Complementary Filter/Pose Complementary Filter ==
  note: Complementary filter
  Rate : Inport
  Correction : Inport  Port=2
  Add4 : Sum  Inputs=-+
  Add6 : Sum  Inputs=+--
  Integrator5 : Integrator
  K_i : Gain  Gain=[0 0 0]
  K_p : Gain  Gain=[0 0 0]
  Rate Transition : RateTransition
  Wrap theta to pi : Subsystem
  Wrap theta to pi1 : Subsystem
  Estimate : Outport
  wires:
  Add4/1 -> Wrap theta to pi1/1(angle in)
  Integrator5/1 -> Wrap theta to pi/1(angle in)
  Correction/1 -> Rate Transition/1
  Add6/1 -> Integrator5/1
  Rate Transition/1 -> Add4/1
  Rate/1 -> Add6/1
  Wrap theta to pi/1(angle out) -> Add4/2, Estimate/1
  Wrap theta to pi1/1(angle out) -> K_p/1

== system sensor_fusion/State Estimation with Complementary Filter/Turn Speed Complementary Filter ==
  note: Complementary filter
  Rate : Inport
  Correction : Inport  Port=2
  Add4 : Sum  Inputs=-+
  Add6 : Sum  Inputs=+--
  Integrator : Integrator
  Integrator5 : Integrator
  K_i : Gain  Gain=0
  K_p : Gain  Gain=0
  Turn Speed Estimate : Scope  NumInputPorts=3
      settings: TimeSpan=10  Title=Turn Speed  ActiveDisplayYMinimum=-0.35854983368522886  ActiveDisplayYMaximum=0.507510766445452  DataLoggingVariableName=ScopeData11
  Estimate : Outport
  wires:
  Add6/1 -> Integrator5/1
  Rate/1 -> Integrator/1, Add6/1
  Correction/1 -> Turn Speed Estimate/2, Add4/1  "Correction"
  Integrator5/1 -> Turn Speed Estimate/3, Estimate/1, Add4/2  "Fused"
  Integrator/1 -> Turn Speed Estimate/1  "Integrated rate"

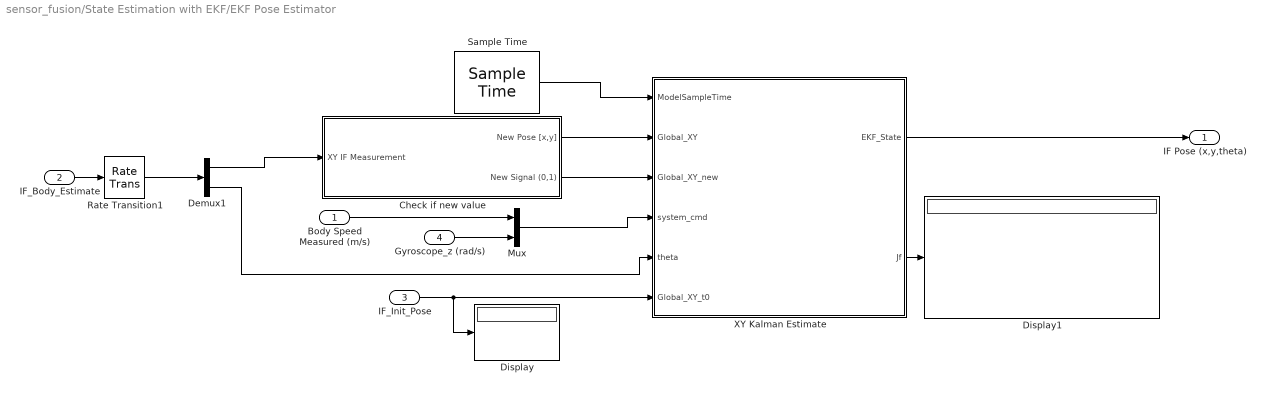
== system sensor_fusion/State Estimation with EKF/EKF Pose Estimator ==
  Body Speed Measured (m/s) : Inport
  IF_Body_Estimate : Inport  Port=2
  IF_Init_Pose : Inport  Port=3
  Gyroscope_z (rad/s) : Inport  Port=4
  Check if new value : Subsystem
  Demux1 : Demux  Outputs=[2,1]
  Display : Display
  Display1 : Display
  Mux : Mux  Inputs=2
  Rate Transition1 : RateTransition
  Sample Time : quarc_library/Sources/Time/Sample Time  Priority=-99  sample_time=qc_get_step_size
  XY Kalman Estimate : MATLAB Function  TreatAsAtomicUnit=on
  IF Pose (x,y,theta) : Outport
  wires:
  Sample Time/1 -> XY Kalman Estimate/1(ModelSampleTime)
  Demux1/1 -> Check if new value/1("XY IF Measurement ")
  IF_Init_Pose/1 -> Display/1, XY Kalman Estimate/6(Global_XY_t0)
  IF_Body_Estimate/1 -> Rate Transition1/1
  Check if new value/1(New Pose [x,y]) -> XY Kalman Estimate/2(Global_XY)
  Check if new value/2(New Signal (0,1)) -> XY Kalman Estimate/3(Global_XY_new)
  XY Kalman Estimate/1(EKF_State) -> IF Pose (x,y,theta)/1
  Body Speed Measured (m/s)/1 -> Mux/1
  Mux/1 -> XY Kalman Estimate/4(system_cmd)
  XY Kalman Estimate/2(Jf) -> Display1/1
  Gyroscope_z (rad/s)/1 -> Mux/2
  Demux1/2 -> XY Kalman Estimate/5(theta)
  Rate Transition1/1 -> Demux1/1

== system sensor_fusion/State Estimation with Complementary Filter/Pose Complementary Filter/Wrap theta to pi ==
  angle in : Inport
  Assignment : Assignment  DiagnosticForDimensions=Warning  IndexOptions=Index vector (dialog)  Indices=3  OutputSizes=1
  Selector1 : Selector  InputPortWidth=3  IndexOptions=Index vector (dialog)  Indices=[3]  OutputSizes=1
  Wrap theta to pi : MATLAB Function  TreatAsAtomicUnit=on
  Wrap theta to pi1 : MATLAB Function  Commented=on  TreatAsAtomicUnit=on
  angle out : Outport
  wires:
  angle in/1 -> Assignment/1, Selector1/1
  Selector1/1 -> Wrap theta to pi/1(u)
  Wrap theta to pi/1(y) -> Assignment/2
  Assignment/1 -> angle out/1

== system sensor_fusion/State Estimation with Complementary Filter/Pose Complementary Filter/Wrap theta to pi1 ==
  angle in : Inport
  Assignment : Assignment  DiagnosticForDimensions=Warning  IndexOptions=Index vector (dialog)  Indices=3  OutputSizes=1
  Selector1 : Selector  InputPortWidth=3  IndexOptions=Index vector (dialog)  Indices=[3]  OutputSizes=1
  Wrap theta to pi : MATLAB Function  TreatAsAtomicUnit=on
  Wrap theta to pi1 : MATLAB Function  Commented=on  TreatAsAtomicUnit=on
  angle out : Outport
  wires:
  Assignment/1 -> angle out/1
  Wrap theta to pi/1(y) -> Assignment/2
  Selector1/1 -> Wrap theta to pi/1(u)
  angle in/1 -> Selector1/1, Assignment/1

== system sensor_fusion/State Estimation with EKF/EKF Pose Estimator/Check if new value ==
  "XY IF Measurement " : Inport
  Detect Change : simulink/Logic and Bit Operations/Detect Change  vinit=0  OutDataTypeStr=boolean
  Memory : Memory
  Norm : quarc_library/Math Operations/Vectors/Norm
      settings: SourceProductName=QUARC Targets
  Rate Transition : RateTransition
  Switch : Switch  Criteria=u2 > Threshold  SaturateOnIntegerOverflow=off  InputSameDT=off
  New Pose [x,y] : Outport
  New Signal (0,1) : Outport  Port=2
  wires:
  "XY IF Measurement "/1 -> Switch/1, Norm/1
  Norm/1 -> Detect Change/1
  Switch/1 -> Rate Transition/1
  Memory/1 -> Switch/3
  Detect Change/1 -> Switch/2, New Signal (0,1)/1
  Rate Transition/1 -> New Pose [x,y]/1, Memory/1

== matlab function sensor_fusion/State Estimation with Complementary Filter/Pose Complementary Filter/Wrap theta to pi1/Wrap theta to pi1 ==
  data: u input; y output
function y = wrap_to_pi(u)
y = mod(u+pi, 2*pi)-pi;

== matlab function sensor_fusion/State Estimation with Complementary Filter/Differential Drive Forward Velocity Kinematics ==
  data: wL input; vForward output; wR input; omega output
function [vForward , omega] = forKin(wL, wR)

% calculate wheel angular velocities
wheelRadius = 3.5*0.0254/2;

vR = wR * wheelRadius;
vL = wL * wheelRadius;

% wheelbase
d=0.3928; 

% calculate wheel linear velocities
vForward = (vR + vL)/2;
omega = (vR - vL)/d;

== matlab function sensor_fusion/Joystick Driver/MATLAB Function ==
  data: u input; N output; S output; E output; W output
function [N, S, E, W] = fcn(u)

N = 0;
S = 0;
E = 0;
W = 0;

switch u
    case 0
        N = 1;
    case 3.142
        S = 1;
    case 4.712
        W = 1;
    case 1.571
        E = 1;
    case 3.927
        S = 1;
        W = 1;
    case 2.356
        S = 1;
        E = 1;
    case 0.7854
        N = 1;
        E = 1;
    case 5.498
        N = 1;
        W = 1;
end

== matlab function sensor_fusion/QBot Hardware/Differential Drive Forward Velocity Kinematics ==
  data: wL input; vC output; wR input; Omega output
function [vC , Omega] = forKin(wL, wR)

% calculate wheel angular velocities
wheelRadius = 3.5*0.0254/2;

vR = wR * wheelRadius;
vL = wL * wheelRadius;

% wheelbase
d=0.3928; 

% calculate wheel linear velocities
vC = (vR + vL)/2;
Omega = (vR - vL)/d;

== matlab function sensor_fusion/Lidar & Localization/Subsample & Correct LiDAR/Adjust for Center of Measurement ==
  data: lidar_position input; ranges input; ranges_c output; angles input; angles_c output
function [ranges_c,angles_c] = correct_lidar(lidar_position, ranges,angles)

% Convert lidar data from polar into cartesian, and add lidar position
% Then convert back into polar coordinates
%-------Replace the following line with your code---------%
ranges_c = ranges;
angles_c = angles./angles;
%---------------------------------------------------------%

end

== matlab function sensor_fusion/State Estimation with Complementary Filter/Pose Complementary Filter/Wrap theta to pi/Wrap theta to pi ==
  data: u input; y output
function y = wrap_to_pi(u)
y = atan2(sin(u), cos(u));

== matlab function sensor_fusion/State Estimation with EKF/Differential Drive Forward Velocity Kinematics ==
  data: wL input; vForward output; wR input; omega output
function [vForward , omega] = forKin(wL, wR)

% calculate wheel angular velocities
wheelRadius = 3.5*0.0254/2;

vR = wR * wheelRadius;
vL = wL * wheelRadius;

% wheelbase
d=0.3928; 

% calculate wheel linear velocities
vForward = (vR + vL)/2;
omega = (vR - vL)/d;

== matlab function sensor_fusion/State Estimation with Complementary Filter/MATLAB Function ==
  data: xSpeed output; ySpeed output; forSpd input; theta input
function [xSpeed,ySpeed] = calculate_xy_speeds(forSpd, theta)

    xSpeed = forSpd*cos(theta);
    ySpeed = forSpd*sin(theta);

end

== matlab function sensor_fusion/State Estimation with Complementary Filter/Pose Complementary Filter/Wrap theta to pi/Wrap theta to pi1 ==
  data: u input; y output
function y = wrap_to_pi(u)
y = mod(u+pi, 2*pi)-pi;

== matlab function sensor_fusion/State Estimation with Complementary Filter/Pose Complementary Filter/Wrap theta to pi1/Wrap theta to pi ==
  data: u input; y output
function y = wrap_to_pi(u)
y = atan2(sin(u), cos(u));

== matlab function sensor_fusion/State Estimation with EKF/EKF Pose Estimator/XY Kalman Estimate ==
  data: ModelSampleTime input; Global_XY input; EKF_State output; Global_XY_new input; system_cmd input; theta input; Global_XY_t0 input; Jf output
function [EKF_State, Jf] = ekf_estimate( ...
    ModelSampleTime, Global_XY, Global_XY_new, ...
    system_cmd, theta, Global_XY_t0)

%% Extended Kalman Filter for a differential-drive robot
%
% State:
%   x = [X;
%        Y;
%        theta]
%
% Control input:
%   system_cmd(1) = linear velocity  v     [m/s]
%   system_cmd(2) = angular velocity omega [rad/s]
%
% Measurement:
%   Global_XY = measured global position [X,Y]
%   theta     = measured global heading


persistent x P 

%% ---------------------------------------------------------------
% Initialization
% ---------------------------------------------------------------
if isempty(x)

    % Initial EKF state obtained from the initial global pose.
    x = [Global_XY_t0(1);
         Global_XY_t0(2);
         theta];

    % Initial state covariance.
    P = 0.01 * eye(3);

    % First call has no elapsed time.
    dt = 0;

    EKF_State = x;
    Jf = eye(3);

    return;
end

%% ---------------------------------------------------------------
% Calculate elapsed time
% ---------------------------------------------------------------
dt = ModelSampleTime;

% Protection against invalid or zero time steps.
if dt <= 0
    dt = eps;
end

%% ---------------------------------------------------------------
% EKF tuning matrices
% ---------------------------------------------------------------

% Process noise covariance.
%
% These values should eventually be tuned based on the uncertainty in
% the wheel velocity / odometry measurements.
Q = 0.0075 * eye(3);

% Measurement covariance.
%
% Ideally X/Y and theta should have individually tuned variances because
% position is measured in metres while theta is measured in radians.
R = 0.001 * eye(3);

% Full pose measurement matrix:
%
%       z = [X;
%            Y;
%            theta]
%
H = eye(3);

I = eye(3);

%% ---------------------------------------------------------------
% Read control input
% ---------------------------------------------------------------
v     = system_cmd(1);
omega = system_cmd(2);

% IMPORTANT:
% Save heading BEFORE performing the motion prediction.
%
% The Jacobian must be evaluated about the state from which the prediction
% was made, not the already predicted heading.
theta_k = x(3);

%% ===============================================================
% EKF PREDICTION
% ===============================================================

% Threshold used to switch between curved and straight motion models.
omegaThreshold = 0.02;

if abs(omega) > omegaThreshold

    %% -----------------------------------------------------------
    % Exact constant-turn-rate differential-drive motion model
    % -----------------------------------------------------------
    %
    % X(k+1) =
    %   X(k) - v/w*sin(theta)
    %        + v/w*sin(theta + w*dt)
    %
    % Y(k+1) =
    %   Y(k) + v/w*cos(theta)
    %        - v/w*cos(theta + w*dt)
    %
    % theta(k+1) =
    %   theta(k) + w*dt
    %

    theta_next = theta_k + omega*dt;

    x_pred = x + ...
        [-(v/omega)*sin(theta_k) ...
          + (v/omega)*sin(theta_next);

          (v/omega)*cos(theta_k) ...
          - (v/omega)*cos(theta_next);

          omega*dt];

    %% Motion-model Jacobian
    %
    % Jf = df/dx
    Jf = ...
        [1, 0, -(v/omega)*cos(theta_k) ...
                + (v/omega)*cos(theta_next);

         0, 1, -(v/omega)*sin(theta_k) ...
                + (v/omega)*sin(theta_next);

         0, 0, 1];

else

    %% -----------------------------------------------------------
    % Straight-line approximation
    % -----------------------------------------------------------
    %
    % This avoids dividing by omega when omega is approximately zero.
    %

    x_pred = x + ...
        [v*cos(theta_k)*dt;
         v*sin(theta_k)*dt;
         omega*dt];

    %% Straight-motion Jacobian
    Jf = ...
        [1, 0, -v*sin(theta_k)*dt;
         0, 1,  v*cos(theta_k)*dt;
         0, 0,  1];
end

% Normalize predicted heading to [-pi, pi].
x_pred(3) = atan2(sin(x_pred(3)), cos(x_pred(3)));

%% ---------------------------------------------------------------
% Predict covariance
% ---------------------------------------------------------------
P_pred = Jf * P * Jf' + Q;

%% ===============================================================
% EKF MEASUREMENT UPDATE
% ===============================================================

if Global_XY_new

    % Global pose measurement.
    z = [Global_XY(1);
         Global_XY(2);
         theta];

    % Innovation:
    %
    %       innovation = measurement - predicted measurement
    %
    innovation = z - H*x_pred;

    % Heading differences must be normalized.
    %
    % Example:
    %   measured = -179 deg
    %   predicted = +179 deg
    %
    % The error should be +2 deg, not -358 deg.
    innovation(3) = atan2( ...
        sin(innovation(3)), ...
        cos(innovation(3)));

    % Innovation covariance.
    S = H*P_pred*H' + R;

    % Kalman gain.
    %
    % Matrix division is preferred to explicitly computing inv(S).
    K = (P_pred * H') / S;

    % Correct state estimate.
    x = x_pred + K*innovation;

    % Normalize corrected heading.
    x(3) = atan2(sin(x(3)), cos(x(3)));

    % Joseph-form covariance update.
    %
    % This is numerically more robust than:
    %
    %       P = (I-K*H)*P_pred;
    %
    P = (I-K*H)*P_pred*(I-K*H)' + K*R*K';

else

    % No global measurement:
    % prediction becomes the current estimate.
    x = x_pred;
    P = P_pred;
end

%% ---------------------------------------------------------------
% EKF output
% ---------------------------------------------------------------
EKF_State = x;

end
